simulink model "ASM_Traffic_V2X_Complete_Model_2"  (R2019a)
settings: Solver=ode1  StartTime=SIM.tstart.v  StopTime=Inf  FixedStep=SIM.StepSize.v  RelTol=1e-3
PostLoadFcn:
  | if any(exist('dsrtsu_mdlpostloadfcn', 'file') ~= 0), dsrtsu_mdlpostloadfcn('Execute', bdroot); end
  | try, asm_mdl_postloadfcn(bdroot, 'UpdateModel', 2200); catch, disp(lasterr); end,
undefined symbols (not defined in the file): _SensorPnts_1, _SensorPnts_13, _SensorPnts_17, _SensorPnts_21, _SensorPnts_25, _SensorPnts_29, _SensorPnts_33, _SensorPnts_37, _SensorPnts_41, _SensorPnts_45, _SensorPnts_49, _SensorPnts_5, _SensorPnts_53, _SensorPnts_57, _SensorPnts_9, _to_, CPT, G5A, ITS, MDL, rad, s_to_rpm, SIM
libraries: simulink x169, ASM_VehicleDynamics_lib x126, ASM_Traffic_lib x83, ASM_Utils_lib x49, mdbs x45, ASM_Environment_lib x17, dspindex x12, dsaV2xLibraryAux x10, dsmpblib x6, dsaV2xAsn1Library x4, dsaV2xLibrary x4, ASM_BrakeHydraulics_lib x4
(part 6 of 36)

== system ASM_Traffic_V2X_Complete_Model_2/MDL/VehicleDynamics/VehicleMovement ==
  F_Aero_CoorSys_V[x;y;z][N] : Inport
  Trq_Aero_CoorSys_V[x;y;z][Nm] : Inport  Port=2
  F_Tire_CoorSys_V[FL,FR,RL,RR][x;y;z][N] : Inport  Port=3
  Trq_Tire_CoorSys_V[FL,FR,RL,RR][x;y;z][Nm] : Inport  Port=4
  Stiffness_z_Tire[FL,FR,RL,RR][N|m] : Inport  Port=5
  w_Wheel[FL,FR,RL,RR][x;y;z][rad|s] : Inport  Port=6
  Trq_Shaft_CoorSys_V[FL,FR,RL,RR][x;y;z][Nm] : Inport  Port=7
  gF_Susp[q1_Front;q2_Front;q1_Rear;q2_Rear][] : Inport  Port=8
  Pos_Wheel[FL,FR,RL,RR][x;y;z][m] : Inport  Port=9
  w_Rel_WheelBody[FL,FR,RL,RR][x y z][rad|s] : Inport  Port=10
  v_Rel_WheelBody[FL,FR,RL,RR][x;y;z][m|s] : Inport  Port=11
  Pos_Vehicle_Init_CoorSys_E[x;y;z][m] : Inport  Port=12
  Angle_V_Init_CoorSys_E[x;y;z][rad] : Inport  Port=13
  Reset[] : Inport  Port=14
  KeepVehiclePosition[0|1] : Inport  Port=15
  gRear_dq_Rear_dt[2x2][] : Inport  Port=16
  gFront_dq_Front_dt[2x2][] : Inport  Port=17
  SuspensionKinematicsRelations_Rear : Inport  Port=18
  SuspensionKinematicsRelations_Front : Inport  Port=19
  F_External_CoorSys_V[x,y,z][N] : Inport  Port=20
  Trq_External_CoorSys_V[x,y,z][Nm] : Inport  Port=21
  Stabilization_F_External[3X6] : Inport  Port=22
  Stabilization_Trq_External[3X6] : Inport  Port=23
  q_dt_Init[:] : Inport  Port=24
  q_Wheel_Init[:] : Inport  Port=25
  ASMSignalCollector : Subsystem
  Bus Selector1 : BusSelector  OutputSignals=Pos_RL_Wheel_dq_Rear[q1;q2][x;y;z][],w_Rel_RL_Wheel_dq_Rear_dt[q1;q2][x;y;z][],Pos_RR_Wheel_dq_Rear[q1;q2][x;y;z][],w_Rel_RR_Wheel_dq_Rear[q1;q2][x;y;z][]
  Bus Selector2 : BusSelector  OutputSignals=Pos_FL_Wheel_dq_Front[q1;q2][x;y;z][],w_Rel_FL_Wheel_dq_Front_dt[q1;q2][x;y;z][],Pos_FR_Wheel_dq_Front[q1;q2][x;y;z][],w_Rel_FR_Wheel_dq_Front[q1;q2][x;y;z][]
  COORDINATE_TRANSFORMATION : ASM_VehicleDynamics_lib/VehicleDynamics/VehicleMovement/COORDINATE_TRANSFORMATION  Tag=ASM_SUBCOMPONENT  StepSize=SIM.StepSize  ASMProperties=struct('Name','COORDINATE_TRANSFORMATION','Version','4.0','Library','ASM_VehicleDynamics_lib')  ASMInstanceName=coordinate_transformation  ASMInstanceID=1
  J : Constant  Value=zeros(3,3)
  MASS_FORCES_AND_TORQUES : ASM_VehicleDynamics_lib/VehicleDynamics/VehicleMovement/MASS_FORCES_AND_TORQUES  Tag=ASM_SUBCOMPONENT  ASMProperties=struct('Name','MASS_FORCES_AND_TORQUES','Version','2.0','Library','ASM_VehicleDynamics_lib')  ASMInstanceName=mass_forces_and_torques  ASMInstanceID=1
  OR : Subsystem
  SENSOR_MOTION : ASM_VehicleDynamics_lib/VehicleDynamics/VehicleMovement/SENSOR_MOTION  Tag=ASM_SUBCOMPONENT  Const_PosVec_Sensor1=MDL.VehicleDynamics.VehicleMovement.SensorMotion.Const_PosVec_Sensor1  Const_PosVec_Sensor2=MDL.VehicleDynamics.VehicleMovement.SensorMotion.Const_PosVec_Sensor2  Const_PosVec_Sensor3=MDL.VehicleDynamics.VehicleMovement.SensorMotion.Const_PosVec_Sensor3  Const_PosVec_Sensor4=MDL.VehicleDynamics.VehicleMovement.SensorMotion.Const_PosVec_Sensor4  ASMProperties=struct('Name','SENSOR_MOTION','Version','4.0','Library','ASM_VehicleDynamics_lib')  ASMInstanceName=sensor_motion  ASMInstanceID=1
  Selector1 : Selector  InputPortWidth=15  IndexOptions=Index vector (dialog)  Indices=[4:15]  OutputSizes=1
  Selector2 : Selector  InputPortWidth=15  IndexOptions=Index vector (dialog)  Indices=[4:15]  OutputSizes=1
  Selector3 : Selector  InputPortWidth=15  IndexOptions=Index vector (dialog)  Indices=[4:15]  OutputSizes=1
  Sw_TestBenchMode[1Vehicle|2TestBench] : Constant
  Terminator : Terminator
  VEHICLE_AND_WHEEL_VELOCITIES : ASM_VehicleDynamics_lib/VehicleDynamics/VehicleMovement/VEHICLE_AND_WHEEL_VELOCITIES  Tag=ASM_SUBCOMPONENT  ASMProperties=struct('Name','VEHICLE_AND_WHEEL_VELOCITIES','Version','1.0','Library','ASM_VehicleDynamics_lib')  ASMInstanceName=vehicle_and_wheel_velocities  ASMInstanceID=1
  VEHICLE_MASS_AND_ADDITIONAL_LOADS : ASM_VehicleDynamics_lib/VehicleDynamics/VehicleMovement/VEHICLE_MASS_AND_ADDITIONAL_LOADS  Tag=ASM_SUBCOMPONENT  Const_m_Vehicle=MDL.VehicleDynamics.Vehicle.Const_m_Vehicle  Const_PosVec_CoG_Vehicle=MDL.VehicleDynamics.Vehicle.Const_PosVec_CoG_Vehicle  Const_Inertia_Tensor_Vehicle=MDL.VehicleDynamics.Vehicle.Const_Inertia_Tensor_Vehicle  Const_m_AddLoad1=MDL.VehicleDynamics.VehicleMovement.AddLoad1.Const_m_AddLoad1  Const_PosVec_CoG_AddLoad1=MDL.VehicleDynamics.VehicleMovement.AddLoad1.Const_PosVec_CoG_AddLoad1  Const_Inertia_Tensor_AddLoad1=MDL.VehicleDynamics.VehicleMovement.AddLoad1.Const_Inertia_Tensor_AddLoad1  Sw_AddLoad1=MDL.VehicleDynamics.VehicleMovement.AddLoad1.Sw_AddLoad1  Const_m_AddLoad2=MDL.VehicleDynamics.VehicleMovement.AddLoad2.Const_m_AddLoad2  Const_PosVec_CoG_AddLoad2=MDL.VehicleDynamics.VehicleMovement.AddLoad2.Const_PosVec_CoG_AddLoad2  Const_Inertia_Tensor_AddLoad2=MDL.VehicleDynamics.VehicleMovement.AddLoad2.Const_Inertia_Tensor_AddLoad2  Sw_AddLoad2=MDL.VehicleDynamics.VehicleMovement.AddLoad2.Sw_AddLoad2  Const_m_AddLoad3=MDL.VehicleDynamics.VehicleMovement.AddLoad3.Const_m_AddLoad3  Const_PosVec_CoG_AddLoad3=MDL.VehicleDynamics.VehicleMovement.AddLoad3.Const_PosVec_CoG_AddLoad3  Const_Inertia_Tensor_AddLoad3=MDL.VehicleDynamics.VehicleMovement.AddLoad3.Const_Inertia_Tensor_AddLoad3  Sw_AddLoad3=MDL.VehicleDynamics.VehicleMovement.AddLoad3.Sw_AddLoad3  Const_m_AddLoad4=MDL.VehicleDynamics.VehicleMovement.AddLoad4.Const_m_AddLoad4  Const_PosVec_CoG_AddLoad4=MDL.VehicleDynamics.VehicleMovement.AddLoad4.Const_PosVec_CoG_AddLoad4  Const_Inertia_Tensor_AddLoad4=MDL.VehicleDynamics.VehicleMovement.AddLoad4.Const_Inertia_Tensor_AddLoad4  Sw_AddLoad4=MDL.VehicleDynamics.VehicleMovement.AddLoad4.Sw_AddLoad4  Const_m_AddLoad5=MDL.VehicleDynamics.VehicleMovement.AddLoad5.Const_m_AddLoad5  Const_PosVec_CoG_AddLoad5=MDL.VehicleDynamics.VehicleMovement.AddLoad5.Const_PosVec_CoG_AddLoad5  Const_Inertia_Tensor_AddLoad5=MDL.VehicleDynamics.VehicleMovement.AddLoad5.Const_Inertia_Tensor_AddLoad5  Sw_AddLoad5=MDL.VehicleDynamics.VehicleMovement.AddLoad5.Sw_AddLoad5  Const_m_AddLoad6=MDL.VehicleDynamics.VehicleMovement.AddLoad6.Const_m_AddLoad6  Const_PosVec_CoG_AddLoad6=MDL.VehicleDynamics.VehicleMovement.AddLoad6.Const_PosVec_CoG_AddLoad6  Const_Inertia_Tensor_AddLoad6=MDL.VehicleDynamics.VehicleMovement.AddLoad6.Const_Inertia_Tensor_AddLoad6  Sw_AddLoad6=MDL.VehicleDynamics.VehicleMovement.AddLoad6.Sw_AddLoad6  ASMProperties=struct('Name','VEHICLE_MASS_AND_ADDITIONAL_LOADS','Version','3.0','Library','ASM_VehicleDynamics_lib')  ASMInstanceName=vehicle_mass_and_additional_loads  ASMInstanceID=1
  VEHICLE_MOTION_CAR : ASM_VehicleDynamics_lib/VehicleDynamics/VehicleMovement/VEHICLE_MOTION_CAR  Tag=ASM_SUBCOMPONENT  StepSize=SIM.StepSize  ASMProperties=struct('Name','VEHICLE_MOTION_CAR','Version','5.0','Library','ASM_VehicleDynamics_lib')  ASMInstanceName=vehicle_motion_car  ASMInstanceID=1
  m : Constant  Value=0
  r_CoG : Constant  Value=[0 0 0]
  ASMSignalBus : Outport
  v_Abs_Vehicle_CoG[x;y;z][m|s] : Outport  Port=2
  RotationMatrix_V_to_E_T[3x3] : Outport  Port=3
  Pos_Wheels_CoorSys_E[FL,FR,RL,RR][x;y;z][m] : Outport  Port=4
  v_Abs_WheelBody_CoorSys_V[FL,FR,RL,RR][x y z][m|s] : Outport  Port=5
  w_Abs_Wheel_CoorSys_V[FL,FR,RL,RR][x,y,z][rad|s] : Outport  Port=6
  F_Gyroscopic[FL,FR,RL,RR][x;y;z][N] : Outport  Port=7
  Trq_Gyroscopic[FL,FR,RL,RR][x;y;z][Nm] : Outport  Port=8
  F_Gravitational[FL,FR,RL,RR][x;y;z][N] : Outport  Port=9
  q_Wheel_dt[q1_Front;q2_Front;q1_Rear;q2_Rear][] : Outport  Port=10
  q_Wheel[q1_Front;q2_Front;q1_Rear;q2_Rear][] : Outport  Port=11
  tag scope: ASMBUS_VehicleDynamics_CoGAndWheelVelocities=global, ASMBUS_VehicleDynamics_CoordinateTransformation=global, ASMBUS_VehicleDynamics_MassForcesAndTorques=global, ASMBUS_VehicleDynamics_SensorMotion=global, ASMBUS_VehicleDynamics_VehicleMass=global, ASMBUS_VehicleDynamics_VehicleMotion=global
  wires:
  m/1 -> VEHICLE_MASS_AND_ADDITIONAL_LOADS/1
  r_CoG/1 -> VEHICLE_MASS_AND_ADDITIONAL_LOADS/2
  J/1 -> VEHICLE_MASS_AND_ADDITIONAL_LOADS/3
  COORDINATE_TRANSFORMATION/5 -> SENSOR_MOTION/6
  q_Wheel_Init[:]/1 -> VEHICLE_MOTION_CAR/32
  q_dt_Init[:]/1 -> VEHICLE_MOTION_CAR/31
  OR/1(Out) -> VEHICLE_MOTION_CAR/1
  KeepVehiclePosition[0|1]/1 -> OR/1(In1)
  Sw_TestBenchMode[1Vehicle|2TestBench]/1 -> VEHICLE_MOTION_CAR/30
  Stabilization_Trq_External[3X6]/1 -> VEHICLE_MOTION_CAR/29
  Stabilization_F_External[3X6]/1 -> VEHICLE_MOTION_CAR/28
  Trq_External_CoorSys_V[x,y,z][Nm]/1 -> VEHICLE_MOTION_CAR/27
  F_External_CoorSys_V[x,y,z][N]/1 -> VEHICLE_MOTION_CAR/26
  Selector3/1 -> F_Gravitational[FL,FR,RL,RR][x;y;z][N]/1
  Selector1/1 -> F_Gyroscopic[FL,FR,RL,RR][x;y;z][N]/1
  Selector2/1 -> Trq_Gyroscopic[FL,FR,RL,RR][x;y;z][Nm]/1
  ASMSignalCollector/1(ASMSignalBus) -> ASMSignalBus/1
  SuspensionKinematicsRelations_Rear/1 -> Bus Selector1/1
  Bus Selector1/4 -> VEHICLE_MOTION_CAR/23  "<w_Rel_RR_Wheel_dq_Rear[q1;q2][x;y;z][]>"
  Bus Selector1/3 -> VEHICLE_MOTION_CAR/22  "<Pos_RR_Wheel_dq_Rear[q1;q2][x;y;z][]>"
  Bus Selector1/2 -> VEHICLE_MOTION_CAR/21  "<w_Rel_RL_Wheel_dq_Rear_dt[q1;q2][x;y;z][]>"
  Bus Selector1/1 -> VEHICLE_MOTION_CAR/20  "<Pos_RL_Wheel_dq_Rear[q1;q2][x;y;z][]>"
  Bus Selector2/4 -> VEHICLE_MOTION_CAR/19  "<w_Rel_FR_Wheel_dq_Front[q1;q2][x;y;z][]>"
  Bus Selector2/3 -> VEHICLE_MOTION_CAR/18  "<Pos_FR_Wheel_dq_Front[q1;q2][x;y;z][]>"
  Bus Selector2/2 -> VEHICLE_MOTION_CAR/17  "<w_Rel_FL_Wheel_dq_Front_dt[q1;q2][x;y;z][]>"
  Bus Selector2/1 -> VEHICLE_MOTION_CAR/16  "<Pos_FL_Wheel_dq_Front[q1;q2][x;y;z][]>"
  SuspensionKinematicsRelations_Front/1 -> Bus Selector2/1
  gRear_dq_Rear_dt[2x2][]/1 -> VEHICLE_MOTION_CAR/25
  gFront_dq_Front_dt[2x2][]/1 -> VEHICLE_MOTION_CAR/24
  Trq_Shaft_CoorSys_V[FL,FR,RL,RR][x;y;z][Nm]/1 -> VEHICLE_MOTION_CAR/9
  Stiffness_z_Tire[FL,FR,RL,RR][N|m]/1 -> VEHICLE_MOTION_CAR/8
  Trq_Aero_CoorSys_V[x;y;z][Nm]/1 -> VEHICLE_MOTION_CAR/7
  F_Aero_CoorSys_V[x;y;z][N]/1 -> VEHICLE_MOTION_CAR/6
  Trq_Tire_CoorSys_V[FL,FR,RL,RR][x;y;z][Nm]/1 -> VEHICLE_MOTION_CAR/5
  F_Tire_CoorSys_V[FL,FR,RL,RR][x;y;z][N]/1 -> VEHICLE_MOTION_CAR/4
  Pos_Wheel[FL,FR,RL,RR][x;y;z][m]/1 -> VEHICLE_MOTION_CAR/3, VEHICLE_AND_WHEEL_VELOCITIES/3, COORDINATE_TRANSFORMATION/2
  gF_Susp[q1_Front;q2_Front;q1_Rear;q2_Rear][]/1 -> VEHICLE_MOTION_CAR/2
  Reset[]/1 -> OR/2(In2), COORDINATE_TRANSFORMATION/1, ASMSignalCollector/1(Reset[])
  VEHICLE_MOTION_CAR/3 -> q_Wheel[q1_Front;q2_Front;q1_Rear;q2_Rear][]/1
  COORDINATE_TRANSFORMATION/4 -> MASS_FORCES_AND_TORQUES/7, SENSOR_MOTION/5
  Angle_V_Init_CoorSys_E[x;y;z][rad]/1 -> COORDINATE_TRANSFORMATION/6
  Pos_Vehicle_Init_CoorSys_E[x;y;z][m]/1 -> COORDINATE_TRANSFORMATION/5
  COORDINATE_TRANSFORMATION/3 -> RotationMatrix_V_to_E_T[3x3]/1
  COORDINATE_TRANSFORMATION/2 -> Pos_Wheels_CoorSys_E[FL,FR,RL,RR][x;y;z][m]/1
  VEHICLE_AND_WHEEL_VELOCITIES/2 -> Terminator/1
  MASS_FORCES_AND_TORQUES/4 -> VEHICLE_MOTION_CAR/13, Selector3/1
  SENSOR_MOTION/1 -> [ASMBUS_VehicleDynamics_SensorMotion]
  VEHICLE_MOTION_CAR/5 -> SENSOR_MOTION/2
  VEHICLE_MOTION_CAR/4 -> SENSOR_MOTION/1
  w_Wheel[FL,FR,RL,RR][x;y;z][rad|s]/1 -> MASS_FORCES_AND_TORQUES/6, VEHICLE_AND_WHEEL_VELOCITIES/6
  v_Rel_WheelBody[FL,FR,RL,RR][x;y;z][m|s]/1 -> MASS_FORCES_AND_TORQUES/5, VEHICLE_AND_WHEEL_VELOCITIES/4
  w_Rel_WheelBody[FL,FR,RL,RR][x y z][rad|s]/1 -> VEHICLE_AND_WHEEL_VELOCITIES/5
  VEHICLE_MOTION_CAR/2 -> q_Wheel_dt[q1_Front;q2_Front;q1_Rear;q2_Rear][]/1
  VEHICLE_MASS_AND_ADDITIONAL_LOADS/2 -> VEHICLE_MOTION_CAR/12, MASS_FORCES_AND_TORQUES/8
  VEHICLE_MASS_AND_ADDITIONAL_LOADS/3 -> VEHICLE_MOTION_CAR/11, MASS_FORCES_AND_TORQUES/9
  VEHICLE_MASS_AND_ADDITIONAL_LOADS/4 -> VEHICLE_MOTION_CAR/10, VEHICLE_AND_WHEEL_VELOCITIES/7
  VEHICLE_MASS_AND_ADDITIONAL_LOADS/1 -> [ASMBUS_VehicleDynamics_VehicleMass]
  MASS_FORCES_AND_TORQUES/1 -> [ASMBUS_VehicleDynamics_MassForcesAndTorques]
  VEHICLE_MOTION_CAR/7 -> VEHICLE_AND_WHEEL_VELOCITIES/1, SENSOR_MOTION/3, COORDINATE_TRANSFORMATION/3
  VEHICLE_MOTION_CAR/6 -> SENSOR_MOTION/4, COORDINATE_TRANSFORMATION/4, MASS_FORCES_AND_TORQUES/4, VEHICLE_AND_WHEEL_VELOCITIES/2
  MASS_FORCES_AND_TORQUES/2 -> VEHICLE_MOTION_CAR/15, Selector2/1
  MASS_FORCES_AND_TORQUES/3 -> VEHICLE_MOTION_CAR/14, Selector1/1
  VEHICLE_AND_WHEEL_VELOCITIES/6 -> MASS_FORCES_AND_TORQUES/3
  VEHICLE_AND_WHEEL_VELOCITIES/4 -> MASS_FORCES_AND_TORQUES/1, v_Abs_WheelBody_CoorSys_V[FL,FR,RL,RR][x y z][m|s]/1
  VEHICLE_AND_WHEEL_VELOCITIES/5 -> MASS_FORCES_AND_TORQUES/2, v_Abs_Vehicle_CoG[x;y;z][m|s]/1
  VEHICLE_AND_WHEEL_VELOCITIES/3 -> w_Abs_Wheel_CoorSys_V[FL,FR,RL,RR][x,y,z][rad|s]/1
  VEHICLE_MOTION_CAR/1 -> [ASMBUS_VehicleDynamics_VehicleMotion]
  VEHICLE_AND_WHEEL_VELOCITIES/1 -> [ASMBUS_VehicleDynamics_CoGAndWheelVelocities]
  COORDINATE_TRANSFORMATION/1 -> [ASMBUS_VehicleDynamics_CoordinateTransformation]

== system ASM_Traffic_V2X_Complete_Model_2/MDLUserInterface/Drivetrain/MDL_DISP ==
  ActiveTransmission : Subsystem
  AutomaticTransmission : Subsystem
  Bus Selector2 : BusSelector  OutputSignals=Crankshaft,Starter,FinalDriveAssembly.Shaft_CF,FinalDriveAssembly.Shaft_CR,FinalDriveAssembly.Shaft_FL,FinalDriveAssembly.Shaft_FR,FinalDriveAssembly.Shaft_RL,FinalDriveAssembly.Shaft_RR,Transmission.ActiveTransmission,Transmission.ManualTransmission,Transmission.AutomaticTransmission
  EngineSpeed : Subsystem
  ManualTransmission : Subsystem
  Shafts : Subsystem
  wires:
  [ASMBUS_Drivetrain] -> Bus Selector2/1
  Bus Selector2/1 -> EngineSpeed/1(Crankshaft)  "<Crankshaft>"
  Bus Selector2/2 -> EngineSpeed/2(Starter)  "<Starter>"
  Bus Selector2/3 -> Shafts/1(Shaft_CF)  "<Shaft_CF>"
  Bus Selector2/4 -> Shafts/2(Shaft_CR)  "<Shaft_CR>"
  Bus Selector2/5 -> Shafts/3(Shaft_FL)  "<Shaft_FL>"
  Bus Selector2/6 -> Shafts/4(Shaft_FR)  "<Shaft_FR>"
  Bus Selector2/7 -> Shafts/5(Shaft_RL)  "<Shaft_RL>"
  Bus Selector2/8 -> Shafts/6(Shaft_RR)  "<Shaft_RR>"
  Bus Selector2/9 -> ActiveTransmission/1(ActiveTrm)  "<ActiveTransmission>"
  Bus Selector2/10 -> ManualTransmission/1(ManTrm)  "<ManualTransmission>"
  Bus Selector2/11 -> AutomaticTransmission/1(AutoTrm)  "<AutomaticTransmission>"

== system ASM_Traffic_V2X_Complete_Model_2/MDLUserInterface/Drivetrain/MDL_PAR ==
  Const_LoadTorque[Nm] : Constant  Value=0
  DRIVETRAIN_VARIANT_SWITCHES : ASM_VehicleDynamics_lib/Drivetrain/DRIVETRAIN_VARIANT_SWITCHES  Tag=ASM_SUBCOMPONENT  SW_Transmission_Mode=MDL.Drivetrain.SW_Transmission_Mode.v  SW_Drivetrain_Mode=MDL.Drivetrain.SW_Drivetrain_Mode.v  ASMProperties=struct('Name','DRIVETRAIN_VARIANT_SWITCHES','Version','4.0','Library','ASM_VehicleDynamics_lib')  ASMInstanceName=drivetrain_variant_switches  ASMInstanceID=1
  Sw_CrankShaft_Reset[0Disabled|1Enabled] : Constant
  Sw_LoadTorque[0MDL|1Constant] : Constant  Value=0
  tag scope: TAG_Drivetrain_Const_LoadTorque=global, TAG_Drivetrain_SW_LoadTorque_Mode=global, TAG_Drivetrain_Sw_CrankShaft_Reset=global
  wires:
  Sw_LoadTorque[0MDL|1Constant]/1 -> [TAG_Drivetrain_SW_LoadTorque_Mode]
  Const_LoadTorque[Nm]/1 -> [TAG_Drivetrain_Const_LoadTorque]
  Sw_CrankShaft_Reset[0Disabled|1Enabled]/1 -> [TAG_Drivetrain_Sw_CrankShaft_Reset]

== system ASM_Traffic_V2X_Complete_Model_2/MDLUserInterface/Drivetrain/MDL_TEST ==

== system ASM_Traffic_V2X_Complete_Model_2/MDLUserInterface/Engine/MDL_DISP ==
  note: Dummy blocks for ControlDesk layout.
      | Might be replaced when simulating virtual vehicles.
  Bus Selector1 : BusSelector  OutputSignals=EngineTorques.Trq_Eff_Engine[Nm],EngineTorques.Trq_Fric_Engine[Nm],EngineTorques.Trq_Ind_Engine[Nm]
  Bus Selector10 : BusSelector  OutputSignals=FuelConsumption.CO2_Emission.CO2_Emission[kg|h],FuelConsumption.CO2_Emission.CO2_Emission_Total[kg],FuelConsumption.Fuel_Consumption[l|h],FuelConsumption.Fuel_Consumption_Total[l],FuelConsumption.mdot_Fuel[g|h],FuelConsumption.b_e[g|kWh],FuelConsumption.Efficiency.eta_Eff_Engine[0_1],FuelConsumption.Efficiency.eta_Ind_Engine[0_1],FuelConsumption.Efficiency.eta_Mechanical_Engine[0_1]
  Bus Selector9 : BusSelector  OutputSignals=VehicleMovement.Velocities.Vehicle.Linear.v_Total_Vehicle[km|h]
  CO2_Emission[kg|100km] : Subsystem
      mask Display: disp('')
  CO2_Emission[kg|100km]_ : Subsystem
  CO2_Emission[kg|h] : Subsystem
      mask Display: disp('')
  CO2_Emission_Total[kg] : Subsystem
      mask Display: disp('')
  CarbonEmission : Scope  NumInputPorts=3
  Efficiency : Scope  NumInputPorts=3
  Engine : Scope  NumInputPorts=3
  FuelConsumption : Scope  NumInputPorts=5
  FuelTank : Constant  Value=0.5
  FuelTank[0|1] : Subsystem
      mask Display: disp('')
  Fuel_Consumption[L|100km] : Subsystem
      mask Display: disp('')
  Fuel_Consumption[L|100km]_ : Subsystem
  Fuel_Consumption[l|h] : Subsystem
      mask Display: disp('')
  Fuel_Consumption_Total[l] : Subsystem
      mask Display: disp('')
  T_Water : Constant
  T_Water[degC] : Subsystem
      mask Display: disp('')
  Terminator : Terminator
  Terminator2 : Terminator
  Trq_Eff_Engine[Nm] : Subsystem
      mask Display: disp('')
  Trq_Fric_Engine[Nm] : Subsystem
      mask Display: disp('')
  Trq_Ind_Engine[Nm] : Subsystem
      mask Display: disp('')
  b_e[g|kWh] : Subsystem
      mask Display: disp('')
  eta_Eff_Engine[0_1] : Subsystem
      mask Display: disp('')
  eta_Ind_Engine[0_1] : Subsystem
      mask Display: disp('')
  eta_Mechanical_Engine[0_1] : Subsystem
      mask Display: disp('')
  mdot_Fuel[g|h] : Subsystem
      mask Display: disp('')
  wires:
  FuelTank/1 -> FuelTank[0|1]/1(In1)
  T_Water/1 -> T_Water[degC]/1(In1)
  FuelTank[0|1]/1(Out1) -> Terminator/1
  T_Water[degC]/1(Out1) -> Terminator2/1
  [ASMBUS_EngineBasic] -> Bus Selector10/1, Bus Selector1/1
  Bus Selector1/1 -> Trq_Eff_Engine[Nm]/1(In1)  "<Trq_Eff_Engine[Nm]>"
  Bus Selector1/2 -> Trq_Fric_Engine[Nm]/1(In1)  "<Trq_Fric_Engine[Nm]>"
  Bus Selector1/3 -> Trq_Ind_Engine[Nm]/1(In1)  "<Trq_Ind_Engine[Nm]>"
  Trq_Eff_Engine[Nm]/1(Out1) -> Engine/1  "Trq_Eff_Engine[Nm]"
  Trq_Fric_Engine[Nm]/1(Out1) -> Engine/2  "Trq_Fric_Engine[Nm]"
  Trq_Ind_Engine[Nm]/1(Out1) -> Engine/3  "Trq_Ind_Engine[Nm]"
  Fuel_Consumption[L|100km]_/1(Fuel_Consumption[l|100km]) -> Fuel_Consumption[L|100km]/1(In1)
  Bus Selector9/1 -> Fuel_Consumption[L|100km]_/1(v_Vehicle[km|h]), CO2_Emission[kg|100km]_/1(v_Vehicle[km|h])  "<v_Total_Vehicle[km|h]>"
  [ASMBUS_VehicleDynamics] -> Bus Selector9/1
  Bus Selector10/3 -> Fuel_Consumption[L|100km]_/2(Fuel_Consumption[l|h]), Fuel_Consumption[l|h]/1(In1)  "<Fuel_Consumption[l|h]>"
  Bus Selector10/1 -> CO2_Emission[kg|100km]_/2(CO2_Emission[kg|h]), CO2_Emission[kg|h]/1(In1)  "<CO2_Emission[kg|h]>"
  CO2_Emission[kg|100km]_/1(CO2_Emission[kg|100km]) -> CO2_Emission[kg|100km]/1(In1)
  Bus Selector10/2 -> CO2_Emission_Total[kg]/1(In1)  "<CO2_Emission_Total[kg]>"
  Bus Selector10/4 -> Fuel_Consumption_Total[l]/1(In1)  "<Fuel_Consumption_Total[l]>"
  Bus Selector10/5 -> mdot_Fuel[g|h]/1(In1)  "<mdot_Fuel[g|h]>"
  Bus Selector10/6 -> b_e[g|kWh]/1(In1)  "<b_e[g|kWh]>"
  Bus Selector10/7 -> eta_Eff_Engine[0_1]/1(In1)  "<eta_Eff_Engine[0_1]>"
  Bus Selector10/8 -> eta_Ind_Engine[0_1]/1(In1)  "<eta_Ind_Engine[0_1]>"
  Bus Selector10/9 -> eta_Mechanical_Engine[0_1]/1(In1)  "<eta_Mechanical_Engine[0_1]>"
  Fuel_Consumption[L|100km]/1(Out1) -> FuelConsumption/1  "Fuel_Conumption[l|100km]"
  CO2_Emission[kg|100km]/1(Out1) -> CarbonEmission/1  "CO2_Emission[kg|100km]"
  eta_Eff_Engine[0_1]/1(Out1) -> Efficiency/1  "eta_Eff_Engine[0_1]"
  eta_Ind_Engine[0_1]/1(Out1) -> Efficiency/2  "eta_Ind_Engine[0_1]"
  eta_Mechanical_Engine[0_1]/1(Out1) -> Efficiency/3  "eta_Mechanical_Engine[0_1]"
  CO2_Emission[kg|h]/1(Out1) -> CarbonEmission/2  "CO2_Emission[kg|h]"
  CO2_Emission_Total[kg]/1(Out1) -> CarbonEmission/3  "CO2_Emission_Total[kg]"
  Fuel_Consumption[l|h]/1(Out1) -> FuelConsumption/2  "Fuel_Consumption[l|h]"
  Fuel_Consumption_Total[l]/1(Out1) -> FuelConsumption/3  "Fuel_Consumption_Total[l]"
  mdot_Fuel[g|h]/1(Out1) -> FuelConsumption/4  "mdot_Fuel[g|h]"
  b_e[g|kWh]/1(Out1) -> FuelConsumption/5  "b_e[g|kWh]"

== system ASM_Traffic_V2X_Complete_Model_2/MDLUserInterface/Engine/MDL_PAR ==

== system ASM_Traffic_V2X_Complete_Model_2/MDLUserInterface/Engine/MDL_TEST ==

== system ASM_Traffic_V2X_Complete_Model_2/MDLUserInterface/Environment/MDL_DISP ==
  Bus Selector1 : BusSelector  OutputSignals=VehicleMovement.Velocities
  Bus Selector2 : BusSelector  OutputSignals=Road,Maneuver,Traffic,Driver
  Driver : Subsystem
  Maneuver : Subsystem
  Road : Subsystem
  Traffic : Subsystem
  wires:
  [ASMBUS_Environment] -> Bus Selector2/1
  Bus Selector2/1 -> Road/1(Road)  "<Road>"
  Bus Selector2/4 -> Driver/1(Driver)  "<Driver>"
  Bus Selector2/2 -> Maneuver/1(Maneuver)  "<Maneuver>"
  [ASMBUS_VehicleDynamics] -> Bus Selector1/1
  Bus Selector1/1 -> Driver/2(Velocities)  "<Velocities>"
  Bus Selector2/3 -> Traffic/1(ASMSignalBus)  "<Traffic>"

== system ASM_Traffic_V2X_Complete_Model_2/MDLUserInterface/Environment/MDL_PAR ==
  BasicRoad : Subsystem
      mask Display: disp('Basic Road')
  CollisionSensor : Subsystem
      mask Display: disp('Collision Sensor')
  Fellow_VehicleLights : Subsystem
      mask Display: disp('Fellow Vehicle Lights')
  MANEUVER_SELECT_SWITCH : ASM_Environment_lib/Environment/Maneuver/MANEUVER_SELECT_SWITCH  Tag=ASM_SUBCOMPONENT  Sw_Maneuver_Select=MDL.Environment.SW_Maneuver_Select.v  ASMProperties=struct('Name','MANEUVER_SELECT_SWITCH','Version','2.0','Library','ASM_Environment_lib')  ASMInstanceName=maneuver_select_switch  ASMInstanceID=1
  ManeuverControl : Subsystem
      mask Display: disp('Maneuver Control')
  ManeuverSettings : Subsystem
      mask Display: disp('Maneuver Settings')
  ManualControl : Subsystem
      mask Display: disp('Manual Control')
  Objects_DataStreams : Subsystem
      mask Display: disp('Objects Data Streams')
  ROAD_SELECT_SWITCH : ASM_Environment_lib/Environment/Road/ROAD_SELECT_SWITCH  Tag=ASM_SUBCOMPONENT  SW_Road_Select=MDL.Environment.SW_Road_Select.v  ASMProperties=struct('Name','ROAD_SELECT_SWITCH','Version','1.0','Library','ASM_Environment_lib')  ASMInstanceName=road_select_switch  ASMInstanceID=1
  SimulationControl : Subsystem
      mask Display: disp('Simulation Control')
  Testbench : Subsystem
      mask Display: disp('Testbench')
  TrafficControl : Subsystem
      mask Display: disp('Traffic Control')
  Vehicle_Inits : Subsystem
      mask Display: disp('Vehicle Inits')

== system ASM_Traffic_V2X_Complete_Model_2/MDLUserInterface/Environment/MDL_TEST ==
